simulink model "quantum"  (R2021b)
settings: Solver=FixedStepAuto  StartTime=0.0  StopTime=20  FixedStep=0.01  RelTol=1e-3
undefined symbols (not defined in the file): A, a1, a2, a3, a4, C, k1, k2, L, w
settings Model: Creator=Roberto  LastModifiedBy=Roberto

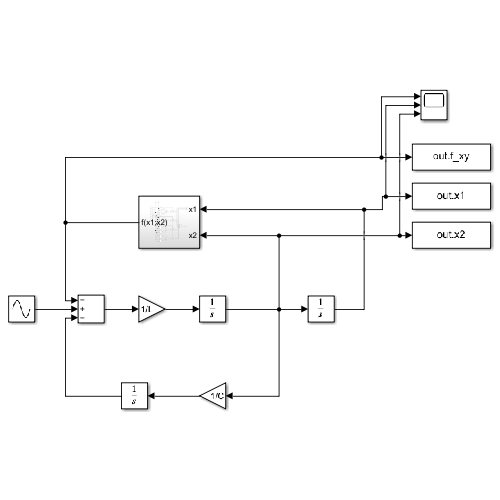
[thumbnail: Simulink's stored preview of the top-level diagram]
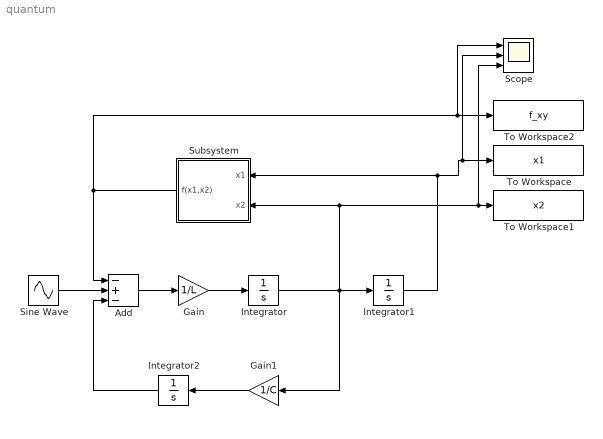
== system quantum ==
  Add : Sum  Inputs=-+-
  Gain : Gain  Gain=1/L
  Gain1 : Gain  Gain=1/C
  Integrator : Integrator
  Integrator1 : Integrator
  Integrator2 : Integrator
  Scope : Scope  NumInputPorts=3
  Sine Wave : Sin  Amplitude=A  Frequency=w  SampleTime=0
  Subsystem : Subsystem
  To Workspace : ToWorkspace  VariableName=x1  SaveFormat=Timeseries  SampleTime=-1
  To Workspace1 : ToWorkspace  VariableName=x2  SaveFormat=Timeseries  SampleTime=-1
  To Workspace2 : ToWorkspace  VariableName=f_xy  SaveFormat=Timeseries  SampleTime=-1
  wires:
  Gain/1 -> Integrator/1
  Add/1 -> Gain/1
  Integrator2/1 -> Add/3
  Gain1/1 -> Integrator2/1
  Integrator/1 -> Integrator1/1, Scope/3, To Workspace1/1, Subsystem/2(x2), Gain1/1
  Integrator1/1 -> Subsystem/1(x1), Scope/2, To Workspace/1
  Subsystem/1(f(x1,x2)) -> Scope/1, To Workspace2/1, Add/1
  Sine Wave/1 -> Add/2

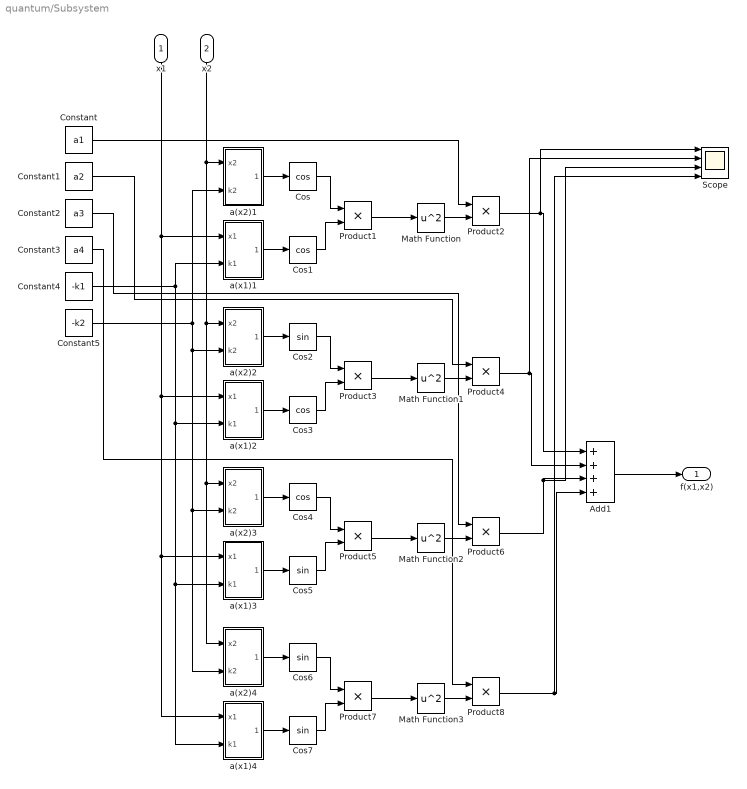
== system quantum/Subsystem ==
  x1 : Inport
  x2 : Inport  Port=2
  Add1 : Sum  Inputs=++++
  Constant : Constant  Value=a1
  Constant1 : Constant  Value=a2
  Constant2 : Constant  Value=a3
  Constant3 : Constant  Value=a4
  Constant4 : Constant  Value=-k1
  Constant5 : Constant  Value=-k2
  Cos{,1,3..4} (4 alike) : Trigonometry  Operator=cos
  Cos{2,5..7} (4 alike) : Trigonometry
  Math Function{,1..3} (4 alike) : Math  Operator=square  SaturateOnIntegerOverflow=on
  Product{1..8} (8 alike) : Product
  Scope : Scope  NumInputPorts=4
  a(x1)1 : Subsystem
  a(x1)2 : Subsystem
  a(x1)3 : Subsystem
  a(x1)4 : Subsystem
  a(x2)1 : Subsystem
  a(x2)2 : Subsystem
  a(x2)3 : Subsystem
  a(x2)4 : Subsystem
  f(x1,x2) : Outport
  wires:
  Constant2/1 -> Product6/1
  x1/1 -> a(x1)1/1(x1), a(x1)4/1(x1), a(x1)3/1(x1), a(x1)2/1(x1)
  Math Function2/1 -> Product6/2
  Constant1/1 -> Product4/1
  Product3/1 -> Math Function1/1
  a(x1)3/1(Out1) -> Cos5/1
  a(x1)2/1(Out1) -> Cos3/1
  Cos2/1 -> Product3/1
  Constant4/1 -> a(x1)3/2(k1), a(x1)4/2(k1), a(x1)2/2(k1), a(x1)1/2(k1)
  Math Function3/1 -> Product8/2
  a(x2)3/1(Out1) -> Cos4/1
  Product5/1 -> Math Function2/1
  Cos5/1 -> Product5/2
  Product1/1 -> Math Function/1
  Product6/1 -> Scope/3, Add1/3
  Constant5/1 -> a(x2)2/2(k2), a(x2)3/2(k2), a(x2)4/2(k2), a(x2)1/2(k2)
  Constant3/1 -> Product8/1
  Math Function/1 -> Product2/2
  Product2/1 -> Scope/1, Add1/1
  Cos/1 -> Product1/1
  Cos4/1 -> Product5/1
  Product8/1 -> Scope/4, Add1/4
  Cos3/1 -> Product3/2
  a(x2)2/1(Out1) -> Cos2/1
  Add1/1 -> f(x1,x2)/1
  Math Function1/1 -> Product4/2
  a(x1)4/1(Out1) -> Cos7/1
  x2/1 -> a(x2)1/1(x2), a(x2)2/1(x2), a(x2)4/1(x2), a(x2)3/1(x2)
  a(x2)1/1(Out1) -> Cos/1
  Constant/1 -> Product2/1
  a(x1)1/1(Out1) -> Cos1/1
  Cos1/1 -> Product1/2
  a(x2)4/1(Out1) -> Cos6/1
  Cos7/1 -> Product7/2
  Product7/1 -> Math Function3/1
  Cos6/1 -> Product7/1
  Product4/1 -> Scope/2, Add1/2

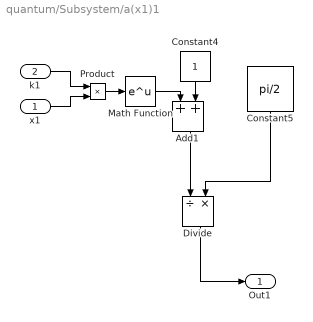
== system quantum/Subsystem/a(x1)1 ==
  x1 : Inport
  k1 : Inport  Port=2
  Add1 : Sum
  Constant4 : Constant
  Constant5 : Constant  Value=pi/2
  Divide : Product  Inputs=/*
  Math Function : Math  SaturateOnIntegerOverflow=on
  Product : Product
  Out1 : Outport
  wires:
  Constant5/1 -> Divide/2
  Add1/1 -> Divide/1
  Math Function/1 -> Add1/1
  Constant4/1 -> Add1/2
  x1/1 -> Product/2
  Divide/1 -> Out1/1
  Product/1 -> Math Function/1
  k1/1 -> Product/1

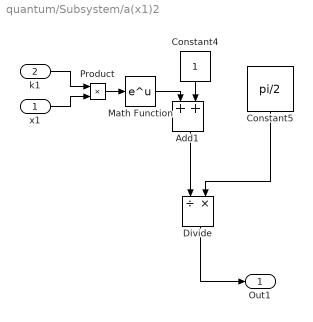
== system quantum/Subsystem/a(x1)2 ==
  x1 : Inport
  k1 : Inport  Port=2
  Add1 : Sum
  Constant4 : Constant
  Constant5 : Constant  Value=pi/2
  Divide : Product  Inputs=/*
  Math Function : Math  SaturateOnIntegerOverflow=on
  Product : Product
  Out1 : Outport
  wires:
  Constant5/1 -> Divide/2
  Add1/1 -> Divide/1
  Math Function/1 -> Add1/1
  Constant4/1 -> Add1/2
  x1/1 -> Product/2
  Divide/1 -> Out1/1
  Product/1 -> Math Function/1
  k1/1 -> Product/1

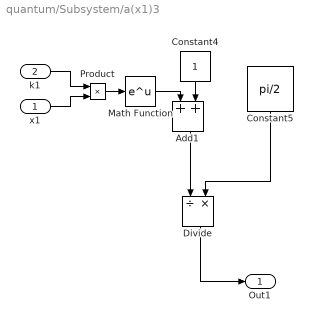
== system quantum/Subsystem/a(x1)3 ==
  x1 : Inport
  k1 : Inport  Port=2
  Add1 : Sum
  Constant4 : Constant
  Constant5 : Constant  Value=pi/2
  Divide : Product  Inputs=/*
  Math Function : Math  SaturateOnIntegerOverflow=on
  Product : Product
  Out1 : Outport
  wires:
  Constant5/1 -> Divide/2
  Add1/1 -> Divide/1
  Math Function/1 -> Add1/1
  Constant4/1 -> Add1/2
  x1/1 -> Product/2
  Divide/1 -> Out1/1
  Product/1 -> Math Function/1
  k1/1 -> Product/1

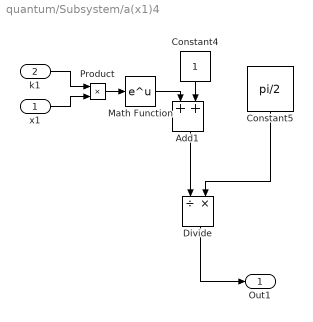
== system quantum/Subsystem/a(x1)4 ==
  x1 : Inport
  k1 : Inport  Port=2
  Add1 : Sum
  Constant4 : Constant
  Constant5 : Constant  Value=pi/2
  Divide : Product  Inputs=/*
  Math Function : Math  SaturateOnIntegerOverflow=on
  Product : Product
  Out1 : Outport
  wires:
  Constant5/1 -> Divide/2
  Add1/1 -> Divide/1
  Math Function/1 -> Add1/1
  Constant4/1 -> Add1/2
  x1/1 -> Product/2
  Divide/1 -> Out1/1
  Product/1 -> Math Function/1
  k1/1 -> Product/1

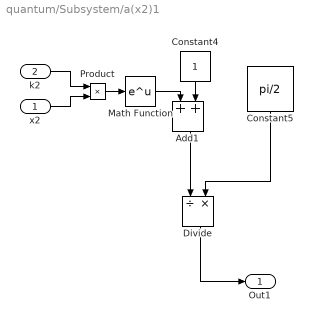
== system quantum/Subsystem/a(x2)1 ==
  x2 : Inport
  k2 : Inport  Port=2
  Add1 : Sum
  Constant4 : Constant
  Constant5 : Constant  Value=pi/2
  Divide : Product  Inputs=/*
  Math Function : Math  SaturateOnIntegerOverflow=on
  Product : Product
  Out1 : Outport
  wires:
  Constant5/1 -> Divide/2
  Add1/1 -> Divide/1
  Math Function/1 -> Add1/1
  Constant4/1 -> Add1/2
  x2/1 -> Product/2
  Divide/1 -> Out1/1
  Product/1 -> Math Function/1
  k2/1 -> Product/1

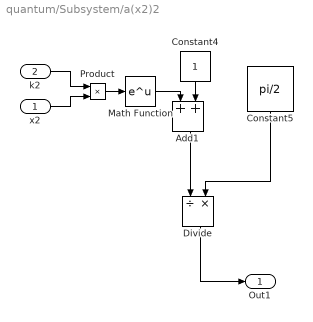
== system quantum/Subsystem/a(x2)2 ==
  x2 : Inport
  k2 : Inport  Port=2
  Add1 : Sum
  Constant4 : Constant
  Constant5 : Constant  Value=pi/2
  Divide : Product  Inputs=/*
  Math Function : Math  SaturateOnIntegerOverflow=on
  Product : Product
  Out1 : Outport
  wires:
  Constant5/1 -> Divide/2
  Add1/1 -> Divide/1
  Math Function/1 -> Add1/1
  Constant4/1 -> Add1/2
  x2/1 -> Product/2
  Divide/1 -> Out1/1
  Product/1 -> Math Function/1
  k2/1 -> Product/1

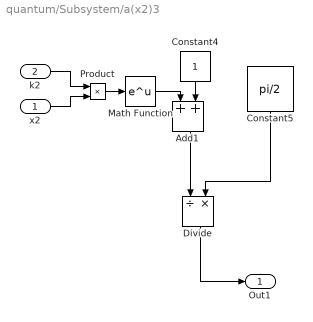
== system quantum/Subsystem/a(x2)3 ==
  x2 : Inport
  k2 : Inport  Port=2
  Add1 : Sum
  Constant4 : Constant
  Constant5 : Constant  Value=pi/2
  Divide : Product  Inputs=/*
  Math Function : Math  SaturateOnIntegerOverflow=on
  Product : Product
  Out1 : Outport
  wires:
  Constant5/1 -> Divide/2
  Add1/1 -> Divide/1
  Math Function/1 -> Add1/1
  Constant4/1 -> Add1/2
  x2/1 -> Product/2
  Divide/1 -> Out1/1
  Product/1 -> Math Function/1
  k2/1 -> Product/1

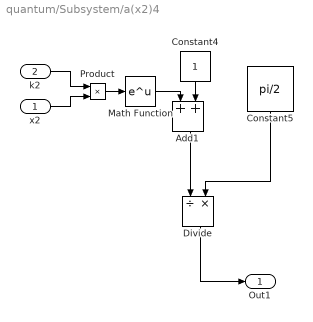
== system quantum/Subsystem/a(x2)4 ==
  x2 : Inport
  k2 : Inport  Port=2
  Add1 : Sum
  Constant4 : Constant
  Constant5 : Constant  Value=pi/2
  Divide : Product  Inputs=/*
  Math Function : Math  SaturateOnIntegerOverflow=on
  Product : Product
  Out1 : Outport
  wires:
  Constant5/1 -> Divide/2
  Add1/1 -> Divide/1
  Math Function/1 -> Add1/1
  Constant4/1 -> Add1/2
  x2/1 -> Product/2
  Divide/1 -> Out1/1
  Product/1 -> Math Function/1
  k2/1 -> Product/1
